simulink model "StateSpace"  (R2023b)
settings: Solver=VariableStepAuto  StartTime=0.0  StopTime=15000  RelTol=1e-3
values from neighbouring files (symbols this model uses):
  designSys = sys0    [LQR2States.m]    (also in LQR2StatesWithDisturb.m; LQR2StatesWithDisturbRecirc.m = sys100)
  K_F = K_ext(1:numInputs, 1:2)    [LQR2States.m]    (also in LQR2StatesWithDisturb.m; LQR2StatesWithDisturbRecirc.m)
  Ki = K_aug(:, n+1:end)    [IntegralActionWithObs.m]    (also in LQR2States.m = K_ext(1:numInputs, 3:4); LQR2StatesWithDisturb.m = K_ext(1:numInputs, 3:4); LQR2StatesWithDisturbRecirc.m = K_ext(1:numInputs, 3:4))
  L = place(A', -C', observer_poles)'    [IntegralActionWithObs.m]    (also in LQR1.m = place(A_new', C_new', p)'; LQR2States.m = place(designSys.A', designSys.C', observer_poles)'; LQR2StatesWithDisturb.m = place(designSys.A', designSys.C', observer_poles)'; LQR2StatesWithDisturbRecirc.m = place(designSys.A', specialC', observer_poles)')
  N_ref = N*v    [LQR2States.m]    (also in LQR2StatesWithDisturb.m; LQR2StatesWithDisturbRecirc.m)
undefined symbols (not defined in the file or in its folder): DiscIntNeverNeededParam, K
settings Model: Creator=jeppe  LastModifiedBy=jeppe

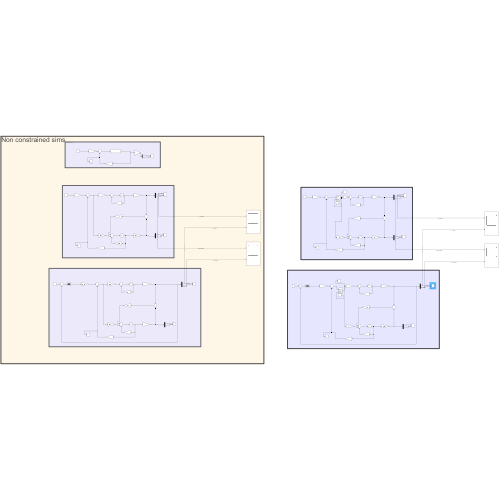
[thumbnail: Simulink's stored preview of the top-level diagram]
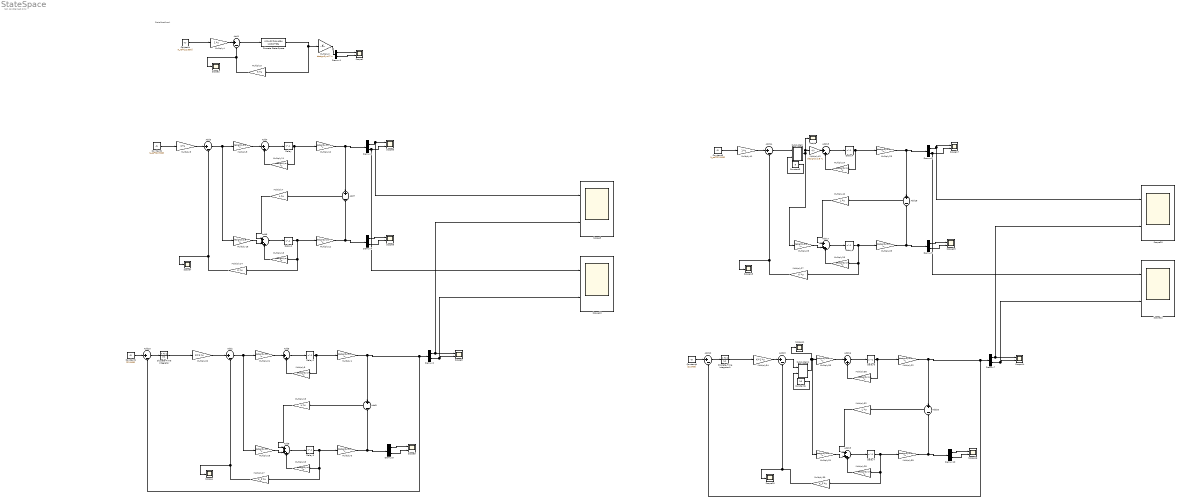
== system StateSpace ==
  note: Non constrained sims
  note: StateFeedback
  Add{1..3,10,12..14} (7 alike) : Sum  Inputs=|+-
  Add{4..5,15..16} (4 alike) : Sum  Inputs=|++
  Add{6,8,17,19} (4 alike) : Sum  Inputs=|+++
  Add{7,9,18,20} (4 alike) : Sum  Inputs=+|-
  Constant : Constant  Value=N_ref*[22;500]
  Constant1 : Constant  Value=[22;500]
  Constant2 : Constant  Value=N_ref*[22;500]
  Constant3 : Constant  Value=5
  Constant4 : Constant  Value=[22;500]
  Constant5 : Constant  Value=N_ref*[22;500]
  Constant6 : Constant  Value=10
  Delay{,1..7} (8 alike) : Delay  DelayLength=1
  Demux{1..5,7..10} (9 alike) : Demux  Outputs=2
  Discrete State-Space : DiscreteStateSpace  A=designSys.A  B=designSys.B  C=[1,0;0,1]  D=designSys.D  SampleTime=15
  Discrete-Time Integrator : DiscreteIntegrator  IntegratorMethod=Integration: Backward Euler  SampleTime=15  ICPrevOutput=DiscIntNeverNeededParam  ICPrevScaledInput=DiscIntNeverNeededParam
  Discrete-Time Integrator1 : DiscreteIntegrator  IntegratorMethod=Integration: Backward Euler  SampleTime=15  ICPrevOutput=DiscIntNeverNeededParam  ICPrevScaledInput=DiscIntNeverNeededParam
  Multiply{1..2,6,10,12,22..23,25,39} (9 alike) : Gain  Gain=designSys.C  Multiplication=Matrix(K*u)
  Multiply{5,11,13,15,24,26,28,38} (8 alike) : Gain  Gain=designSys.A  Multiplication=Matrix(K*u)
  Multiply14 : Gain  Gain=K  Multiplication=Matrix(K*u)
  Multiply{9,16,18,21,29,31,35,42} (8 alike) : Gain  Gain=designSys.B  Multiplication=Matrix(K*u)
  Multiply17 : Gain  Gain=K_F  Multiplication=Matrix(K*u)
  Multiply{7,19,32,40} (4 alike) : Gain  Gain=L  Multiplication=Matrix(K*u)
  Multiply20 : Gain  Gain=Ki*1  Multiplication=Matrix(K*u)
  Multiply27 : Gain  Gain=K  Multiplication=Matrix(K*u)
  Multiply3 : Gain  Gain=K  Multiplication=Matrix(K*u)
  Multiply30 : Gain  Gain=K_F  Multiplication=Matrix(K*u)
  Multiply34 : Gain  Gain=Ki*1  Multiplication=Matrix(K*u)
  Multiply4 : Gain  Multiplication=Matrix(K*u)
  Multiply41 : Gain  Multiplication=Matrix(K*u)
  Multiply8 : Gain  Multiplication=Matrix(K*u)
  Scope{,2,4,7,11,15,18} (7 alike) : Scope
  Scope{1,3,5..6,8..10,12,14,16..17,19..20} (13 alike) : Scope  NumInputPorts=2
  Subsystem : Subsystem
  Subsystem1 : Subsystem
  wires:
  Multiply3/1 -> Scope2/1, Add1/2
  Demux1/1 -> Scope1/1  "T"
  Demux1/2 -> Scope1/2  "CO2"
  Multiply2/1 -> Demux1/1  "y"
  Constant/1 -> Multiply4/1
  Multiply4/1 -> Add1/1
  Discrete State-Space/1 -> Multiply3/1, Multiply2/1
  Add1/1 -> Discrete State-Space/1
  Constant2/1 -> Multiply8/1
  Multiply8/1 -> Add3/1
  Multiply9/1 -> Add4/1
  Add4/1 -> Delay/1
  Multiply11/1 -> Add4/2
  Delay/1 -> Multiply11/1, Multiply10/1
  Demux3/1 -> Scope9/1, Scope6/1  "T_Feedback"
  Demux3/2 -> Scope10/1, Scope6/2  "CO2_Feedback"
  Multiply10/1 -> Add7/1, Demux3/1
  Add6/1 -> Delay1/1
  Multiply14/1 -> Add3/2, Scope7/1
  Add3/1 -> Multiply16/1, Multiply9/1
  Demux4/2 -> Scope8/2  "CO2"
  Multiply12/1 -> Add7/2, Demux4/1
  Demux4/1 -> Scope8/1  "T"
  Delay1/1 -> Multiply12/1, Multiply14/1, Multiply13/1
  Add7/1 -> Multiply7/1
  Multiply7/1 -> Add6/1
  Multiply13/1 -> Add6/3
  Multiply16/1 -> Add6/2
  Add5/1 -> Delay2/1
  Multiply5/1 -> Add5/2
  Add2/1 -> Multiply18/1, Multiply21/1
  Multiply20/1 -> Add2/1
  Delay2/1 -> Multiply5/1, Multiply1/1
  Multiply21/1 -> Add5/1
  Multiply19/1 -> Add8/1
  Add9/1 -> Multiply19/1
  Multiply18/1 -> Add8/2
  Multiply17/1 -> Add2/2, Scope4/1
  Add8/1 -> Delay3/1
  Demux5/1 -> Scope5/1  "T"
  Delay3/1 -> Multiply6/1, Multiply17/1, Multiply15/1
  Demux2/2 -> Scope10/2, Scope3/2  "CO2_integral"
  Demux2/1 -> Scope9/2, Scope3/1  "T__integral"
  Multiply15/1 -> Add8/3
  Demux5/2 -> Scope5/2  "CO2"
  Multiply6/1 -> Add9/2, Demux5/1
  Discrete-Time Integrator/1 -> Multiply20/1
  Constant1/1 -> Add10/1
  Add10/1 -> Discrete-Time Integrator/1
  Multiply1/1 -> Add9/1, Add10/2, Demux2/1
  Add15/1 -> Delay4/1
  Constant5/1 -> Multiply41/1
  Add18/1 -> Multiply40/1
  Multiply23/1 -> Add18/1, Demux8/1
  Multiply24/1 -> Add15/2
  Multiply41/1 -> Add14/1
  Delay4/1 -> Multiply24/1, Multiply23/1
  Multiply40/1 -> Add17/1
  Multiply29/1 -> Add17/2
  Multiply27/1 -> Add14/2, Scope18/1
  Add17/1 -> Delay5/1
  Delay5/1 -> Multiply25/1, Multiply27/1, Multiply26/1
  Delay7/1 -> Multiply39/1, Multiply30/1, Multiply28/1
  Multiply30/1 -> Add13/2, Scope15/1
  Multiply31/1 -> Add19/2
  Add20/1 -> Multiply32/1
  Demux10/2 -> Scope16/2  "CO2"
  Multiply32/1 -> Add19/1
  Multiply35/1 -> Add16/1
  Demux9/1 -> Scope19/1  "T"
  Add13/1 -> Subsystem1/1(signals)
  Multiply38/1 -> Add16/2
  Demux9/2 -> Scope19/2  "CO2"
  Demux7/1 -> Scope20/2, Scope14/1  "T__integral"
  Add16/1 -> Delay6/1
  Demux8/2 -> Scope12/1, Scope17/2  "CO2_Feedback"
  Demux8/1 -> Scope20/1, Scope17/1  "T_Feedback"
  Multiply22/1 -> Add20/1, Add12/2, Demux7/1
  Multiply34/1 -> Add13/1
  Multiply26/1 -> Add17/3
  Add12/1 -> Discrete-Time Integrator1/1
  Constant4/1 -> Add12/1
  Demux7/2 -> Scope12/2, Scope14/2  "CO2_integral"
  Demux10/1 -> Scope16/1  "T"
  Delay6/1 -> Multiply38/1, Multiply22/1
  Multiply25/1 -> Add18/2, Demux9/1
  Discrete-Time Integrator1/1 -> Multiply34/1
  Multiply39/1 -> Add20/2, Demux10/1
  Add19/1 -> Delay7/1
  Multiply28/1 -> Add19/3
  Constant3/1 -> Subsystem/2(T_AO)
  Multiply42/1 -> Add15/1
  Subsystem/1(Out1) -> Scope/1, Multiply42/1, Multiply29/1
  Add14/1 -> Subsystem/1(signals)
  Constant6/1 -> Subsystem1/2(T_AO)
  Subsystem1/1(Out1) -> Scope11/1, Multiply31/1, Multiply35/1

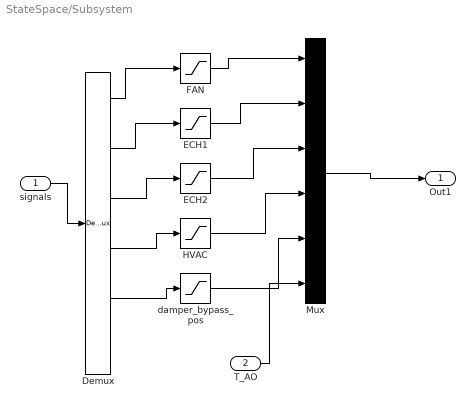
== system StateSpace/Subsystem ==
  signals : Inport
  T_AO : Inport  Port=2
  Demux : Demux  Outputs=6
  ECH1 : Saturate  UpperLimit=100  LowerLimit=0
  ECH2 : Saturate  UpperLimit=100  LowerLimit=0
  FAN : Saturate  UpperLimit=100  LowerLimit=0
  HVAC : Saturate  UpperLimit=100  LowerLimit=-100
  Mux : Mux  Inputs=6
  damper_bypass_pos : Saturate  UpperLimit=100  LowerLimit=0
  Out1 : Outport
  wires:
  signals/1 -> Demux/1
  Demux/1 -> FAN/1
  Demux/2 -> ECH1/1
  Demux/3 -> ECH2/1
  Demux/4 -> HVAC/1
  Demux/5 -> damper_bypass_pos/1
  FAN/1 -> Mux/1
  ECH1/1 -> Mux/2
  ECH2/1 -> Mux/3
  HVAC/1 -> Mux/4
  damper_bypass_pos/1 -> Mux/5
  T_AO/1 -> Mux/6
  Mux/1 -> Out1/1

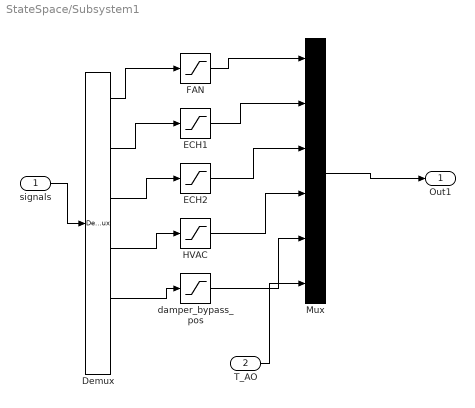
== system StateSpace/Subsystem1 ==
  signals : Inport
  T_AO : Inport  Port=2
  Demux : Demux  Outputs=6
  ECH1 : Saturate  UpperLimit=100  LowerLimit=0
  ECH2 : Saturate  UpperLimit=100  LowerLimit=0
  FAN : Saturate  UpperLimit=100  LowerLimit=0
  HVAC : Saturate  UpperLimit=100  LowerLimit=-100
  Mux : Mux  Inputs=6
  damper_bypass_pos : Saturate  UpperLimit=100  LowerLimit=0
  Out1 : Outport
  wires:
  signals/1 -> Demux/1
  Demux/1 -> FAN/1
  Demux/2 -> ECH1/1
  Demux/3 -> ECH2/1
  Demux/4 -> HVAC/1
  Demux/5 -> damper_bypass_pos/1
  FAN/1 -> Mux/1
  ECH1/1 -> Mux/2
  ECH2/1 -> Mux/3
  HVAC/1 -> Mux/4
  damper_bypass_pos/1 -> Mux/5
  T_AO/1 -> Mux/6
  Mux/1 -> Out1/1
